simulink model "modulation_plots"  (R2022a)
settings: Solver=VariableStepAuto  StartTime=0.0  StopTime=15  RelTol=1e-3
libraries: neuromorphic_blocks x5
settings Model: Creator=chris  LastModifiedBy=chris

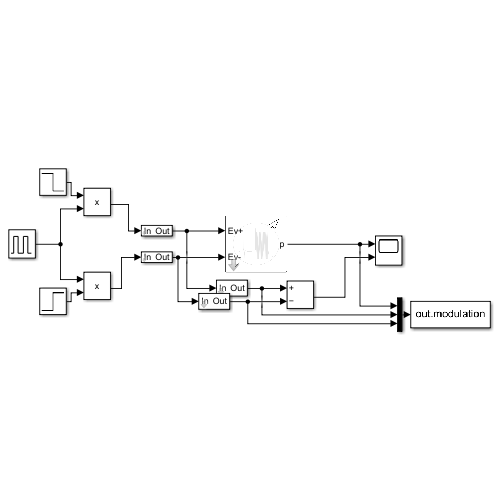
[thumbnail: Simulink's stored preview of the top-level diagram]
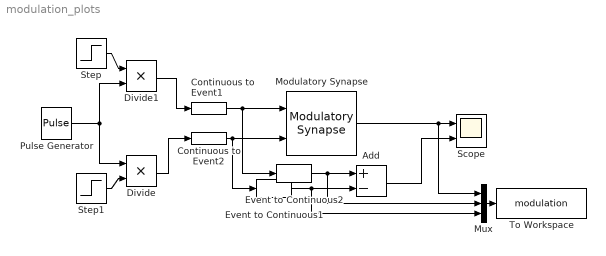
== system modulation_plots ==
  Add : Sum  Inputs=+-
  Continuous to Event1 : neuromorphic_blocks/Events Transmission Blocks/Continuous to Event  thresh=0.5
      settings: SourceProductName=Neuromorphic Toolbox
  Continuous to Event2 : neuromorphic_blocks/Events Transmission Blocks/Continuous to Event  thresh=0.5
      settings: SourceProductName=Neuromorphic Toolbox
  Divide : Product  Inputs=**
  Divide1 : Product  Inputs=**
  Event to Continuous1 : neuromorphic_blocks/Events Transmission Blocks/Event to Continuous  gain=1
      settings: SourceProductName=Neuromorphic Toolbox
  Event to Continuous2 : neuromorphic_blocks/Events Transmission Blocks/Event to Continuous  gain=1
      settings: SourceProductName=Neuromorphic Toolbox
  Modulatory Synapse : neuromorphic_blocks/Neural Blocks/Modulatory Synapse  base_val=0  gsyn_pos_source=Internal  gsyn_pos=5  gsyn_neg_source=Internal  gsyn_neg=5  timescale=0.004  rel_timescale=3000  input=Events  dsyn_pos=5  dsyn_neg=5  msyn_pos=1  msyn_neg=1
      settings: SourceProductName=Neuromorphic Toolbox
  Mux : Mux  Inputs=3
  Pulse Generator : DiscretePulseGenerator  PulseType=Time based  Amplitude=20  Period=0.5  PulseWidth=2  PhaseDelay=0.25
  Scope : Scope  NumInputPorts=2
  Step : Step  Time=4  Before=1  After=0  SampleTime=0
  Step1 : Step  Time=6  SampleTime=0
  To Workspace : ToWorkspace  VariableName=modulation  SaveFormat=Structure With Time  SampleTime=-1
  wires:
  Modulatory Synapse/1 -> Mux/1, Scope/1
  Divide/1 -> Continuous to Event2/1
  Pulse Generator/1 -> Divide1/2, Divide/1
  Step1/1 -> Divide/2
  Step/1 -> Divide1/1
  Divide1/1 -> Continuous to Event1/1
  Add/1 -> Scope/2
  Mux/1 -> To Workspace/1
  Continuous to Event1/1 -> Event to Continuous2/1, Modulatory Synapse/1
  Continuous to Event2/1 -> Event to Continuous1/1, Modulatory Synapse/2
  Event to Continuous1/1 -> Mux/3, Add/2
  Event to Continuous2/1 -> Mux/2, Add/1
